simulink model "imcpendel2"  (R2022b)
settings: Solver=daessc  StartTime=0.0  StopTime=10.0  RelTol=1e-3
values from neighbouring files (symbols this model uses):
  A = eval(A)    [pendulum1.m]
  B = eval(B)    [pendulum1.m]
  C = [1 0]    [pendulum1.m]
  D = [0]    [pendulum1.m]
  G_star_filter = G_star_stable*G_filter    [pendulum1.m]
  xR = [pi; 0]    [pendulum1.m]
libraries: dspsrcs4 x1
settings Model: Creator=mluser  LastModifiedBy=mluser

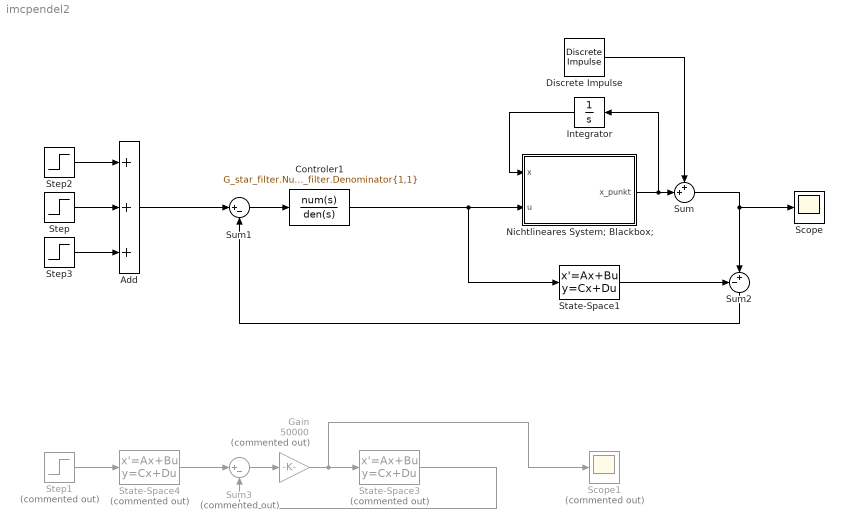
== system imcpendel2 ==
  Add : Sum  Inputs=+++
  Controler1 : TransferFcn  Numerator=G_star_filter.Numerator{1,1}  Denominator=G_star_filter.Denominator{1,1}
  Discrete Impulse : dspsrcs4/Discrete  Impulse  Delay=0  SampleTime=1  FrameSample=1  OutputFrames=off  dataType=double  isSigned=on  wordLen=16  udDataType=sfix(16)  fracBitsMode=Best precision  numFracBits=15  OutDataTypeStr=double  LastOutDataTypeStr=double
  Gain : Gain  Commented=on  Gain=50000
  Integrator : Integrator  InitialCondition=xR
  Nichtlineares System; Blackbox; : MATLAB Function
  Scope : Scope
  Scope1 : Scope  Commented=on
  State-Space1 : StateSpace  A=A  B=B  C=C  D=D  InitialCondition=0
  State-Space3 : StateSpace  Commented=on  A=A  B=B  C=C  D=D  InitialCondition=0
  State-Space4 : StateSpace  Commented=on  A=A  B=B  C=C  D=D  InitialCondition=0
  Step : Step  Time=2  Before=1  After=-1  SampleTime=0
  Step1 : Step  Commented=on  SampleTime=0
  Step2 : Step  SampleTime=0
  Step3 : Step  Time=3  Before=-1  SampleTime=0
  Sum : Sum  Inputs=++|
  Sum1 : Sum  Inputs=|+-
  Sum2 : Sum  Inputs=-+|
  Sum3 : Sum  Commented=on  Inputs=|+-
  wires:
  Controler1/1 -> State-Space1/1, Nichtlineares System; Blackbox;/2(u)
  Sum/1 -> Scope/1, Sum2/2
  Discrete Impulse/1 -> Sum/1
  State-Space1/1 -> Sum2/1
  Sum1/1 -> Controler1/1
  Sum2/1 -> Sum1/2
  State-Space3/1 -> Sum3/2
  Step1/1 -> State-Space4/1
  State-Space4/1 -> Sum3/1
  Gain/1 -> Scope1/1, State-Space3/1
  Sum3/1 -> Gain/1
  Add/1 -> Sum1/1
  Step/1 -> Add/2
  Step3/1 -> Add/3
  Step2/1 -> Add/1
  Nichtlineares System; Blackbox;/1(x_punkt) -> Integrator/1, Sum/2
  Integrator/1 -> Nichtlineares System; Blackbox;/1(x)

== matlab function imcpendel2/Nichtlineares System; Blackbox; ==
  data: x input; x_punkt output; u input
function x_punkt  = fcn(x, u)
x1_punkt = x(2); 
x2_punkt = -sin(x(1)) + u;

x_punkt = [x1_punkt; x2_punkt];
